simulink model "Vehicle_dynamics_Radar_OnlyYaw_2021"  (R2021a)
settings: Solver=FixedStepAuto  StartTime=0.0  StopTime=inf  RelTol=1e-3
values from neighbouring files (symbols this model uses):
  A = 3*3    (= 9)    [Configuration_onlyYaw.m]    (also in test_sim_20000Ep_v2_dist.mat; test_sim_20000Ep_v2_onlyYaw.mat; test_sim_25000Ep_v2_dist.mat; test_sim_25000Ep_v3_onlyYaw.mat)
  alpha = 1e-3    (= 0.001)    [Configuration_onlyYaw.m]
  d = A*N*nCells    (= 699840)    [Configuration_onlyYaw.m]    (also in test_sim_20000Ep_v2_dist.mat; test_sim_20000Ep_v2_onlyYaw.mat; test_sim_25000Ep_v2_dist.mat; test_sim_25000Ep_v3_onlyYaw.mat)
  egoID = 1    [Configuration_onlyYaw.m]    (also in test_sim_20000Ep_v2_dist.mat; test_sim_20000Ep_v2_onlyYaw.mat; test_sim_25000Ep_v2_dist.mat; test_sim_25000Ep_v3_onlyYaw.mat)
  epsilon = 1e-1    (= 0.1)    [Configuration_onlyYaw.m]
  frontDistCG = 3.7    [Configuration_onlyYaw.m]    (also in test_sim_20000Ep_v2_dist.mat; test_sim_20000Ep_v2_onlyYaw.mat; test_sim_25000Ep_v2_dist.mat; test_sim_25000Ep_v3_onlyYaw.mat)
  gamma = 0.9    [Configuration_onlyYaw.m]
  gridvx = [-2.8 -2.75555555556 -2.71111111111 -2.66666666667 -2.62222222222 -2.57777777778 -2.53333333333 -2.48888888889 -2.44444444444 -2.4 -2 -1.95555555556 ... (70 elements, 10x7)]    [test_sim_20000Ep_v2_dist.mat]    (also in test_sim_20000Ep_v2_onlyYaw.mat; test_sim_25000Ep_v2_dist.mat; test_sim_25000Ep_v3_onlyYaw.mat; test_sim_30000Ep_v4_onlyYaw.mat)
  gridvy = [-28 -27.3777777778 -26.7555555556 -26.1333333333 -25.5111111111 -24.8888888889 -24.2666666667 -23.6444444444 -23.0222222222 -22.4 -20 -19.3777777778 ... (70 elements, 10x7)]    [test_sim_20000Ep_v2_dist.mat]    (also in test_sim_20000Ep_v2_onlyYaw.mat; test_sim_25000Ep_v2_dist.mat; test_sim_25000Ep_v3_onlyYaw.mat; test_sim_30000Ep_v4_onlyYaw.mat)
  gridx = [-5 -4.94444444444 -4.88888888889 -4.83333333333 -4.77777777778 -4.72222222222 -4.66666666667 -4.61111111111 -4.55555555556 -4.5 0 0.0555555555556 ... (70 elements, 10x7)]    [test_sim_20000Ep_v2_dist.mat]    (also in test_sim_20000Ep_v2_onlyYaw.mat; test_sim_25000Ep_v2_dist.mat; test_sim_25000Ep_v3_onlyYaw.mat; test_sim_30000Ep_v4_onlyYaw.mat)
  gridy = [0.4 0.453333333333 0.506666666667 0.56 0.613333333333 0.666666666667 0.72 0.773333333333 0.826666666667 0.88 2 2.05333333333 ... (70 elements, 10x7)]    [test_sim_20000Ep_v2_dist.mat]    (also in test_sim_20000Ep_v2_onlyYaw.mat; test_sim_25000Ep_v2_dist.mat; test_sim_25000Ep_v3_onlyYaw.mat; test_sim_30000Ep_v4_onlyYaw.mat)
  gridyaw = [-126 -122.4 -118.8 -115.2 -111.6 -108 -104.4 -100.8 -97.2 -93.6 -90 -86.4 ... (70 elements, 10x7)]    [test_sim_20000Ep_v2_dist.mat]    (also in test_sim_20000Ep_v2_onlyYaw.mat; test_sim_25000Ep_v2_dist.mat; test_sim_25000Ep_v3_onlyYaw.mat; test_sim_30000Ep_v4_onlyYaw.mat)
  lambda = 0.8    [Configuration_onlyYaw.m]
  lb_angSt = -900    [Configuration_onlyYaw.m]    (also in test_sim_20000Ep_v2_dist.mat; test_sim_20000Ep_v2_onlyYaw.mat; test_sim_25000Ep_v2_dist.mat; test_sim_25000Ep_v3_onlyYaw.mat)
  lbvx = -2    [Configuration_onlyYaw.m]    (also in test_sim_20000Ep_v2_dist.mat; test_sim_20000Ep_v2_onlyYaw.mat; test_sim_25000Ep_v2_dist.mat; test_sim_25000Ep_v3_onlyYaw.mat)
  lbvy = -20    [Configuration_onlyYaw.m]    (also in test_sim_20000Ep_v2_dist.mat; test_sim_20000Ep_v2_onlyYaw.mat; test_sim_25000Ep_v2_dist.mat; test_sim_25000Ep_v3_onlyYaw.mat)
  lbx = 0    [Configuration_onlyYaw.m]    (also in test_sim_20000Ep_v2_dist.mat; test_sim_20000Ep_v2_onlyYaw.mat; test_sim_25000Ep_v2_dist.mat; test_sim_25000Ep_v3_onlyYaw.mat)
  lby = 2    [Configuration_onlyYaw.m]    (also in test_sim_20000Ep_v2_dist.mat; test_sim_20000Ep_v2_onlyYaw.mat; test_sim_25000Ep_v2_dist.mat; test_sim_25000Ep_v3_onlyYaw.mat)
  lbyaw = -90    [Configuration_onlyYaw.m]    (also in script_verificaAddestramento.m; script_verificaAddestramento_AllComp.m; test_sim_20000Ep_v2_dist.mat; test_sim_20000Ep_v2_onlyYaw.mat)
  leftDistCG = 0.9    [Configuration_onlyYaw.m]    (also in test_sim_20000Ep_v2_dist.mat; test_sim_20000Ep_v2_onlyYaw.mat; test_sim_25000Ep_v2_dist.mat; test_sim_25000Ep_v3_onlyYaw.mat)
  M = 5    [Configuration_onlyYaw.m]    (also in test_sim_20000Ep_v2_dist.mat; test_sim_20000Ep_v2_onlyYaw.mat; test_sim_25000Ep_v2_dist.mat; test_sim_25000Ep_v3_onlyYaw.mat)
  N = 10    [Configuration_onlyYaw.m]    (also in test_sim_20000Ep_v2_dist.mat; test_sim_20000Ep_v2_onlyYaw.mat; test_sim_25000Ep_v2_dist.mat; test_sim_25000Ep_v3_onlyYaw.mat)
  passo_steerang = 180    [Configuration_onlyYaw.m]    (also in test_sim_20000Ep_v2_dist.mat; test_sim_20000Ep_v2_onlyYaw.mat; test_sim_25000Ep_v2_dist.mat; test_sim_25000Ep_v3_onlyYaw.mat)
  passo_v = 0.5    [Configuration_onlyYaw.m]    (also in test_sim_20000Ep_v2_dist.mat; test_sim_20000Ep_v2_onlyYaw.mat; test_sim_25000Ep_v2_dist.mat; test_sim_25000Ep_v3_onlyYaw.mat)
  retroDistCG = 1    [Configuration_onlyYaw.m]    (also in test_sim_20000Ep_v2_dist.mat; test_sim_20000Ep_v2_onlyYaw.mat; test_sim_25000Ep_v2_dist.mat; test_sim_25000Ep_v3_onlyYaw.mat)
  s = [x_0;-y_0;0;0;-yaw_0]    [script_verificaAddestramento.m]    (also in script_verificaAddestramento_AllComp.m = [x_0;-y_0;0;0;0])
  safetyDist = 0.5    [Configuration_onlyYaw.m]    (also in script_verificaAddestramento_AllComp.m = 0.3; test_sim_20000Ep_v2_dist.mat; test_sim_20000Ep_v2_onlyYaw.mat; test_sim_25000Ep_v2_dist.mat)
  Ts = 0.1    [Configuration_onlyYaw.m]    (also in test_sim_20000Ep_v2_dist.mat; test_sim_20000Ep_v2_onlyYaw.mat; test_sim_25000Ep_v2_dist.mat; test_sim_25000Ep_v3_onlyYaw.mat)
  ub_angSt = 900    [Configuration_onlyYaw.m]    (also in test_sim_20000Ep_v2_dist.mat; test_sim_20000Ep_v2_onlyYaw.mat; test_sim_25000Ep_v2_dist.mat; test_sim_25000Ep_v3_onlyYaw.mat)
  ubvx = 2    [Configuration_onlyYaw.m]    (also in test_sim_20000Ep_v2_dist.mat; test_sim_20000Ep_v2_onlyYaw.mat; test_sim_25000Ep_v2_dist.mat; test_sim_25000Ep_v3_onlyYaw.mat)
  ubvy = 20    [Configuration_onlyYaw.m]    (also in test_sim_20000Ep_v2_dist.mat; test_sim_20000Ep_v2_onlyYaw.mat; test_sim_25000Ep_v2_dist.mat; test_sim_25000Ep_v3_onlyYaw.mat)
  ubx = 25    [Configuration_onlyYaw.m]    (also in test_sim_20000Ep_v2_dist.mat; test_sim_20000Ep_v2_onlyYaw.mat; test_sim_25000Ep_v2_dist.mat; test_sim_25000Ep_v3_onlyYaw.mat)
  uby = 10    [Configuration_onlyYaw.m]    (also in test_sim_20000Ep_v2_dist.mat; test_sim_20000Ep_v2_onlyYaw.mat; test_sim_25000Ep_v2_dist.mat; test_sim_25000Ep_v3_onlyYaw.mat)
  ubyaw = 90    [Configuration_onlyYaw.m]    (also in script_verificaAddestramento.m; script_verificaAddestramento_AllComp.m; test_sim_20000Ep_v2_dist.mat; test_sim_20000Ep_v2_onlyYaw.mat)
  x_0 = 7*rand+7    [Configuration_onlyYaw.m]    (also in script_verificaAddestramento.m = s(1); script_verificaAddestramento_AllComp.m = s(1))
  y_0 = -(0.7*rand+8.5)    [Configuration_onlyYaw.m]    (also in script_verificaAddestramento.m = -s(2); script_verificaAddestramento_AllComp.m = -s(2))
  yaw_0 = deg2rad(65*rand + 5)    [Configuration_onlyYaw.m]    (also in script_verificaAddestramento.m; script_verificaAddestramento_AllComp.m = 0)
undefined symbols (not defined in the file or in its folder): deg, driving, rad
libraries: drivingscenarioandsensors x17, simulink_extras x2, sim3dlib x1, sim3dautolib x1, aerolibconvert2 x1, vehdynlibsteering x1, autolibshared x1
(part 6 of 6)

== matlab function Vehicle_dynamics_Radar_OnlyYaw_2021/Vehicle/MATLAB Function ==
  data: yaw input; yaw_limit output
function yaw_limit = fcn(yaw)

if(yaw > 360)
    yaw_limit = yaw - 360;

elseif(yaw < -360)
     yaw_limit = yaw + 360;
else
    yaw_limit = yaw;
end

end

== matlab function Vehicle_dynamics_Radar_OnlyYaw_2021/Scenario Simulation/Pack Ego Actor ==
  data: pos input; a output Bus: BusActors1Actors size=1; vel input; yaw input; yawRate input; egoID input
function a = packEgo(pos,vel,yaw,yawRate,egoID)
% Pack ego information into a single ego actor bus
%
% Imoprtant note:
% Output is a bus of type BusActorsActors. This is the same bus used by the
% Scenario Reader to output an individual actor. If you change the
% output bus name of Scenario Reader change the output bus name here
% as well by clicking on 'Edit Data' in the menu above.

a = struct(...
    'ActorID',egoID,...
    'Position', [pos(1) pos(2) 0], ...
    'Velocity', [vel(1) vel(2) 0], ...
    'Roll', 0, ...
    'Pitch', 0, ...
    'Yaw', yaw, ...
    'AngularVelocity', [0 0 yawRate]);

== matlab function Vehicle_dynamics_Radar_OnlyYaw_2021/RL_Block_SARSA_ET ==
  settings: updateMethod=DISCRETE  sampleTime=Ts
  data: a_v output [..200]; s input; a2 input; w input; z input; a_steer output; sp input; r input; isTerminal input; w_agg output; st output; z output; stop output; gridx parameter; gridy parameter; gridvx parameter; gridvy parameter; M parameter; N parameter; epsilon parameter; gamma parameter; alpha parameter; A parameter; d parameter; gridyaw parameter; lambda parameter
function [a_v, a_steer, w_agg, st, z, stop] = RL_Block(s, a2, w, z, sp, r, isTerminal, gridx, gridy, gridvx, gridvy, M, N, epsilon, gamma, alpha, A, d, gridyaw, lambda)

coder.extrinsic('assignin') % altrimenti devo usare toWorkspace

% a = [a1;a2] vect colonna con [(1/2/3);(1/2/3)] 
% come gestisco agg parametri w

%steps = steps + 1; % così mostriamo num passi

stop = 0;

% mi serve stato attuale e stato successivo
% creare consistenza tra stato precedente e successivo
a = sub2ind([3 3], a2(1), a2(2));
ae = a;
x = get_features(s, a, gridx, gridy, gridvx, gridvy, gridyaw, M, N, A, d); % features stato attuale
%[sp, r,isTerminal] = dynamics_mountain_car(s, a, lbx, ubx, lbv, ubv); % questo lo prendo da input da modello simulink
if isTerminal
    delta = r - w'*x;
    %assignin("base", "w", w_agg)
    stop = 1;
else                        % da epsilon li devo passare come parameti
    ap = eps_greedy(sp, w, epsilon, gridx, gridy, gridvx, gridvy, gridyaw, M, N, A, d); % azione success
    xp = get_features(sp, ap, gridx, gridy, gridvx, gridvy, gridyaw, M, N, A, d); % features stato success
    delta = r + gamma*w'*xp - w'*x;
    ae = ap;
end
z = gamma*lambda*z + x;
w_agg = w + alpha*delta*z;

if isTerminal
    assignin("base", "w", w_agg)
end
st = sp; % aggiorno              mi manca riferimento ad azione precedente caso isTerminal
%a_v = 0;
[b1,b2] = ind2sub([3 3],ae);

% [1 2 3] vanno mappati su -1,0, con (-2)

if(b1 == 1)
    a_v = 1;
elseif(b1 == 2)
    a_v = 2;
else
    a_v = 3;
end

if(b2 == 1)
    a_steer = 1;
elseif(b2 == 2)
    a_steer = 2;
else
    a_steer = 3;
end

%[a_v,a_steer] = ind2sub([3 3],ae);
%a_v = ones(1,1);
%a_v = b1;
%a_steer = b2;
% cos' mi dava errore di dimensione variabile

%assignin("base", "az_1", b1);

end



%%%%%%%%%%%%%%%%%%%%%%%%%%%%%%%%%%%%%%%%%%%%%%%%%%
%              FUNZIONI AUSILIARE
%%%%%%%%%%%%%%%%%%%%%%%%%%%%%%%%%%%%%%%%%%%%%%%%%%

% Funzione che mi restituisce l'azione epsgreedy da scegliere

function a = eps_greedy(s, w, eps, gridx, gridy, gridvx, gridvy, gridyaw, M, N, A, d)

if rand < eps   % azione random
    a = randi(A); % da 1 a 9 se uso indice
else
    q = zeros(A, 1);
    for a = 1:A  % valuto tutte le azioni che posso prendere
        q(a) = w'*get_features(s, a, gridx, gridy, gridvx, gridvy, gridyaw, M, N, A, d); % approsimazione della funz qualità
    end        % pesi per vett features
    a = find(q == max(q), 1, 'first'); % scelgo quella con funz qualità massima
end
end


function x = get_features(s, a, gridx, gridy, gridvx, gridvy, gridyaw, M, N, A, d)

%coder.extrinsic('assignin')

% numero celle, +1 perchè ne ho aggiunta una
%nCells = (M + 1)^4; % dimensione features per una cella
%d = A*N*nCells; % dimensione vettore pesi da aggiornare
x = zeros(d, 1);
% va modificaro sta dimension var
for ii = 1 : N
    xxx = gridx(ii, :);
    yyy = gridy(ii, :);
    vxvxvx = gridvx(ii, :);
    vyvyvy = gridvy(ii, :);
    yawyawyaw = gridyaw(ii, :);
    % capire in quale cella mi trovo, trovo indice lungo x e lungo y
    ix = find(s(1) >= xxx(1:end-1) & s(1) <= xxx(2:end), 1, 'first');
    iy = find(s(2) >= yyy(1:end-1) & s(2) <= yyy(2:end), 1, 'first');
    ivx = find(s(3) >= vxvxvx(1:end-1) & s(3) <= vxvxvx(2:end), 1, 'first');
    ivy = find(s(4) >= vyvyvy(1:end-1) & s(4) <= vyvyvy(2:end), 1, 'first');
    iyaw = find(s(5) >= yawyawyaw(1:end-1) & s(5) <= yawyawyaw(2:end), 1, 'first');

    % a_ind = sub2ind([3 3],a(1),a(2)); non serve gli passo indice poi da
    % indice a azione quando la uso in dinamica
    % dato doppia dim dell'azione devo subind anche a ???

    % debug
    %pippo = struct('ix',{ix},'iy', {iy},'ivx', {ivx},'ivy', {ivy},'ii', {ii},'a', {a},'s', {s});
    %assignin("base","pippo",pippo);
    ind = sub2ind([M + 1, M + 1, M + 1, M + 1, M + 1, N, A], ix, iy, ivx, ivy, iyaw, ii, a);

    x(ind) = 1; % valore corrispondente alla cella
    % vett features ha un 1 per ogni griglia
end
end

== matlab function Vehicle_dynamics_Radar_OnlyYaw_2021/Reward ==
  data: sp output; next_state input; RadR input; RadF input; RadSx input; RadDx input; camL_L input; camF_L input; camR_L input; r output; isTerminal output; safetyDist parameter; leftDistCG parameter; frontDistCG parameter; retroDistCG parameter; ubx parameter; lbx parameter; uby parameter; lby parameter; ubyaw parameter; lbyaw parameter
% sensori camera hanno difficoltà con ostacoli ravvicinati -> provare radar
function [sp , r, isTerminal] = reward(next_state, RadR, RadF, RadSx, RadDx, camL_L, camF_L, camR_L, safetyDist, leftDistCG, frontDistCG, retroDistCG,ubx, lbx, uby, lby, ubyaw, lbyaw)

% isTerminal quadno crash, quando fuori da ambiente -> r = r - 1000
% isTerminal qunado raggiungo distanza limite dal bordo -> r = 0
% altrimenti r = r - 1

% CG centro asse posteriore

sp = next_state;
%lateral_offset = 1.13;

% controllo posizione non fuori dai limiti (next_state = [x y vx vy])
% limiti ambiente statici, definirli come parametri da workspace
% if((next_state(1) < 0) || (next_state(1) > 25) || (next_state(2) < -10) || (next_state(2) > 10))
%     
%     %fatti cosi sto considerando il centro ma la mia macchina ha delle dimensioni e anche orientamento yaw
%     % se considero misure CG alla fine sto considerando spazio più grande
%     % 
%     r = -1000;
%     isTerminal = 1;
%     return
% end

%fatti cosi sto considerando il centro ma la mia macchina ha delle dimensioni e anche orientamento yaw
% se considero misure CG alla fine sto considerando spazio più grande
if((next_state(1) < lbx) )% || (next_state(1) > 25) || (next_state(2) < -10) || (next_state(2) > 10))
    sp(1) = lbx;
    r = -1000;
    isTerminal = 1;
    return
elseif(next_state(1) > ubx)
    sp(1) = ubx;
    r = -1000;                 % questi numeri vanno sostituiti con i parametri da workspace
    isTerminal = 1;
    return
elseif(next_state(2) < lby)
    sp(2) = lby;
    r = -1000;              % posizione su CG, dovrei calcolare con yaw effettiva dimesione fuori spazio operativo
    isTerminal = 1;
    return
elseif(next_state(2) > uby)
    sp(2) = uby;
    r = -1000;
    isTerminal = 1;
    return
end
% controllo su yaw
if(next_state(5) > ubyaw )
    sp(5) = ubyaw;
    r = -1000;
    isTerminal = 1;
    return
elseif(next_state(5) < lbyaw )
    sp(5) = lbyaw;
    r = -1000;
    isTerminal = 1;
    return
end

%%%%%%%%%%%%%%%%%%%%%%%%%%%%%%%%%%%%%%%%%%%%%%%%%%%%%%%%%%%%%%%%%%%%%%%%%%%
% Per misure sensori verificare distanza da CG
% Sistema di riferimento centrato e fissato nel CG del veicolo
% front e retro(neg) lungo x, lateral lungo y -> misure da considerare
% abs sulle misure
%%%%%%%%%%%%%%%%%%%%%%%%%%%%%%%%%%%%%%%%%%%%%%%%%%%%%%%%%%%%%%%%%%%%%%%%%%%
% per ogni cam ho una serie di detection

% CONTROLLO CRASH  questo lo faccio per ultimo
% utilizzo abs sulle misure mi interessa val assoluto
% Object detection sensore non rileva oggetto non mi ritorna cella, control
% dimensioni veicolo diatnze da CG

% FRONT CRASH
%camF.Detections(i).Measurement(1) % x 
%camF.Detections(i).Measurement(2) % y
i = 1;
while(RadF.Detections(i).Measurement(1) ~= 0) % posizione ritornata va triangolata ???
    % Front controllo su x
    if((abs(RadF.Detections(i).Measurement(1)) - frontDistCG) < safetyDist)
        r = -1000;
        isTerminal = 1;
        return
    end
    i = i + 1;
end 

% RETRO CRASH
i = 1;
while(RadR.Detections(i).Measurement(1) ~= 0) % posizione ritornata va triangolata ???
    % Front controllo su x
    if((abs(RadR.Detections(i).Measurement(1)) - retroDistCG) < safetyDist)
        r = -1000;
        isTerminal = 1;
        return
    end
    i = i + 1;
end 

%LEFT CRASH
i = 1;
while(RadSx.Detections(i).Measurement(2) ~= 0) % posizione ritornata va triangolata ???
    % Front controllo su x
    if((abs(RadSx.Detections(i).Measurement(2)) - leftDistCG) < safetyDist)
        r = -1000;
        isTerminal = 1;
        return
    end
    i = i + 1;
end

%RIGHT CRASH
i = 1;
while(RadDx.Detections(i).Measurement(2) ~= 0) % posizione ritornata va triangolata ???
    % Front controllo su x
    if((abs(RadDx.Detections(i).Measurement(2)) - leftDistCG) < safetyDist)
        r = -1000;
        isTerminal = 1;
        return
    end
    i = i + 1;
end

% Controllo sulle 3 cam la lane dist
% aznche qui devo togliere distanza fissa CG dalla cam che rileva
lateral_offset = camL_L.LaneBoundaries(1).LateralOffset;

if(isnan(lateral_offset))
    lateral_offset = camR_L.LaneBoundaries(1).LateralOffset;
    if(isnan(lateral_offset))
        lateral_offset = camF_L.LaneBoundaries(1).LateralOffset;
        if(isnan(lateral_offset))
%%%%%%%%%%%%%%%%%%%%%%%%%%%%%%%%%%%%%%%%%%%%%%%%%%%%%%%%%%%%%%%%%%%%%%%%%%            
            lateral_offset = 1; % utilizzo lect precedente                  % SISTEMARE QUI PROB Nan 
%%%%%%%%%%%%%%%%%%%%%%%%%%%%%%%%%%%%%%%%%%%%%%%%%%%%%%%%%%%%%%%%%%%%%%%%%%            
        end
    end
end

% CONTROLLO STATO TERMINALE arrivo a dist min dal bordo
% successivame controllo se vado oltre la linea
%if( (abs(lateral_offset) - leftDistCG) < safetyDist + 0.2 
yaw_calc = abs(sp(5));

%if (((abs(lateral_offset) - leftDistCG) <= 1))% && (yaw_calc <= 10) )

% problema qui con primo valore di lateral offset, mi fa terminare ->
% trovare SOLUZIONE
if(((abs(lateral_offset) - leftDistCG) <= 0) || ((abs(lateral_offset) - leftDistCG) > 3))
    r = -1000;
    isTerminal = 1;
    return
end

if(yaw_calc <= 10)
    r = 0;
    isTerminal = 1;
    return
end


%problema se auto gira e legge linea dall'altra parte controllo yaw vlong
%controllo diff posizioni e vedo in che direzione si muove


%Proviamo singola camera laterale con misura da CG
% successivamente proveremo due camere posizionate sulle ruote

%r = -1 - abs(lateral_offset);% - yaw_calc/10;
r = -yaw_calc ;
isTerminal = 0;

== matlab function Vehicle_dynamics_Radar_OnlyYaw_2021/debug_objDet ==
  data: u input; y output; o input; y1 output; y2 output; y3 output
function [y, y1,y2,y3] = fcn(u,o)

%y = u.LaneBoundaries(1).LateralOffset;
%y = size(o.Detections(1).Measurement);

%y = u.LaneBoundaries(1).LateralOffset;
%y1 = u.LaneBoundaries(2).LateralOffset;
%y2 = u.LaneBoundaries(3).LateralOffset;
%y3 = u.LaneBoundaries(4).LateralOffset;
%if(o.Detections(1).Measurement == zeros(1,6))
%    y = 555;
%end
 y = size(o.Detections);
 y1 = o.Detections(1).Measurement;
 y2 = o.Detections(2).Measurement;
 y3 = o.Detections(13).Measurement;


% detection nmero elementi rilevati
% controllo tutti quelli diversi da 6 zeri , no detection tutte zero
%y1= 1;
